simulink model "controller_model_lab_5_R2015"  (R2015a)
settings: Solver=ode5  StartTime=0.0  StopTime=10.0  RelTol=1e-3
values from neighbouring files (symbols this model uses):
  A = [3.98792656502 1 0 0 0 0 -5.81855146071 0 1 0 0 0 ... (36 elements, 6x6)]    [controller_params.mat]    (also in model_params.mat)
  B = [1 0 0 0 0 0]    [controller_params.mat]    (also in model_params.mat)
  C = [-0.000624151634985 0.000754210232314 -7.15793729404e-05 0 0 0]    [controller_params.mat]    (also in model_params.mat)
  D = 0    [controller_params.mat]    (also in model_params.mat)
  DenFilt = [1 -1.6 0.64]    [controller_params.mat]    (also in controller_script.m = poly([alpha alpha]); controller_script_lab_5.m = poly([alpha alpha]))
  kb = compute_strain_constant('plot_collected_data', true, 'plot_selected_data', true)    [compute_constants.m]    (also in compute_strain_constant.m = P(1); controller_params.mat = -7.77292031464; model_params.mat = -7.77292031464)
  Ki_int = -9.9585416323e-05    [controller_params.mat]    (also in controller_script.m = K_int(n_states+1); controller_script_lab_5.m = K_int(n_states+1))
  kp = compute_potentiometer_constant('plot_collected_data', true, 'plot_selected_data', true)    [compute_constants.m]    (also in compute_potentiometer_constant.m = P(1); controller_params.mat = 37.3897251534; model_params.mat = 37.3897251534)
  Kx = [0.00571392119727 -0.0170575156897 0.0161429525348 -0.00224203892548 -0.00421804098625 0.00166256586868]    [controller_params.mat]
  Kx_int = [0.00830854997744 -0.0247918532179 0.023451299358 -0.00325101448541 -0.00612843419234 0.00241434428957]    [controller_params.mat]    (also in controller_script.m = K_int(1:n_states); controller_script_lab_5.m = K_int(1:n_states))
  M = [3543.77501475 3419.31647418 3291.64386704 3161.08265286 3028.02589994 2892.93065581]    [controller_params.mat]
  Nbar = 0.0315325549195    [controller_params.mat]    (also in controller_script.m = Nu + Kx*Nx; controller_script_lab_5.m = Nu + Kx*Nx)
  NumFilt = 0.04    [controller_params.mat]    (also in controller_script.m; controller_script_lab_5.m)
  Ts = 0.001    [controller_params.mat]    (also in controller_script.m; controller_script_lab_5.m)
  x_init = [0 0 0 0 0 0]    [controller_params.mat]    (also in controller_script.m = zeros(n_states, 1); controller_script_lab_5.m = zeros(n_states, 1))
undefined symbols (not defined in the file or in its folder): National_Instruments, PCI
libraries: sldrtlib x3
settings Model: SimulationMode=external  CovHtmlReporting=off  Creator=Alunos  LastModifiedBy=ayesh
settings HardwareCC: ProdBitPerPointer=64  ProdLargestAtomicFloat=Float  ProdIntDivRoundTo=Zero  ProdEndianess=LittleEndian  ProdHWDeviceType=Specified  TargetIntDivRoundTo=Zero  TargetEndianess=LittleEndian  TargetHWDeviceType=Intel->x86/Pentium
settings RTWCC: Description=Simulink Desktop Real-Time  SystemTargetFile=rtwin.tlc  TemplateMakefile=rtwin.tmf  RTWCompilerOptimization=on
settings CodeAppCC: MaxIdLength=95
settings RTWinTargetCC: TargetPreCompLibLocation=C:\Program Files\Polyspace\R2021a\toolbox\sldrt\lib\win64  UseToolchainInfoCompliant=off  ExtModeMexFile=sldrtext

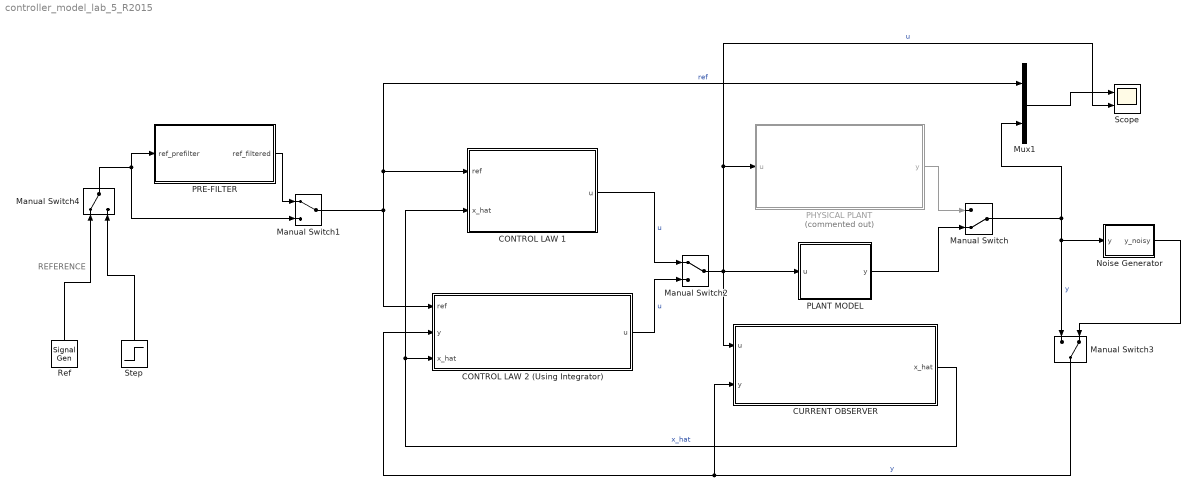
== system controller_model_lab_5_R2015 ==
  note: REFERENCE
  CONTROL LAW 1 : Subsystem
  CONTROL LAW 2 (Using Integrator) : Subsystem
  CURRENT OBSERVER : Subsystem
  Manual Switch : ManualSwitch  CurrentSetting=0
  Manual Switch1 : ManualSwitch
  Manual Switch2 : ManualSwitch
  Manual Switch3 : ManualSwitch  CurrentSetting=0
  Manual Switch4 : ManualSwitch
  Mux1 : Mux  Inputs=2
  Noise Generator : Subsystem
  PHYSICAL PLANT : Subsystem  Commented=on
  PLANT MODEL : Subsystem
  PRE-FILTER : Subsystem
  Ref : SignalGenerator  WaveForm=square  Amplitude=60  Frequency=0.2
  Scope : Scope  NumInputPorts=2
      settings: TimeRange=auto  ShowLegends=on  MaxDataPoints=50000  SaveName=ScopeData  YMin=-75.69471~-4.25511  YMax=75.52983~4.2968  SampleTime=-1
  Step : Step  Time=2  After=30  SampleTime=Ts
  wires:
  Manual Switch2/1 -> Scope/2, PHYSICAL PLANT/1(u), CURRENT OBSERVER/1(u), PLANT MODEL/1(u)  "u"
  Mux1/1 -> Scope/1
  Manual Switch1/1 -> Mux1/1, CONTROL LAW 1/1(ref), CONTROL LAW 2 (Using Integrator)/1(ref)  "ref"
  Manual Switch/1 -> Manual Switch3/1, Noise Generator/1(y), Mux1/2  "y"
  Manual Switch3/1 -> CONTROL LAW 2 (Using Integrator)/2(y), CURRENT OBSERVER/2(y)  "y"
  CURRENT OBSERVER/1(x_hat) -> CONTROL LAW 1/2(x_hat), CONTROL LAW 2 (Using Integrator)/3(x_hat)  "x_hat"
  PLANT MODEL/1(y) -> Manual Switch/2
  PHYSICAL PLANT/1(y) -> Manual Switch/1
  CONTROL LAW 2 (Using Integrator)/1(u) -> Manual Switch2/2  "u"
  CONTROL LAW 1/1(u) -> Manual Switch2/1  "u"
  Noise Generator/1(y_noisy) -> Manual Switch3/2
  Ref/1 -> Manual Switch4/1
  Step/1 -> Manual Switch4/2
  Manual Switch4/1 -> Manual Switch1/2, PRE-FILTER/1(ref_prefilter)
  PRE-FILTER/1(ref_filtered) -> Manual Switch1/1

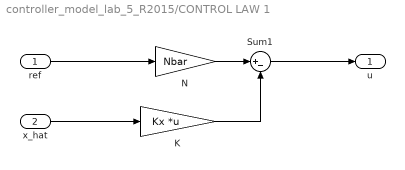
== system controller_model_lab_5_R2015/CONTROL LAW 1 ==
  ref : Inport
  x_hat : Inport  Port=2
  K : Gain  Gain=Kx  Multiplication=Matrix(K*u)
  N : Gain  Gain=Nbar
  Sum1 : Sum  Inputs=|+-
  u : Outport
  wires:
  K/1 -> Sum1/2
  Sum1/1 -> u/1
  N/1 -> Sum1/1
  ref/1 -> N/1
  x_hat/1 -> K/1

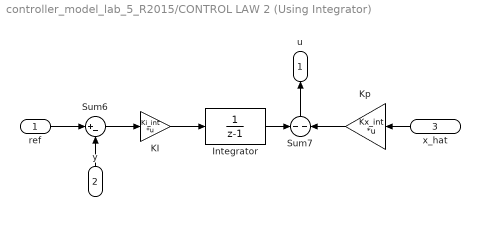
== system controller_model_lab_5_R2015/CONTROL LAW 2 (Using Integrator) ==
  ref : Inport
  y : Inport  Port=2
  x_hat : Inport  Port=3
  Integrator : DiscreteTransferFcn  Denominator=[1 -1]  SampleTime=Ts
  KI : Gain  Gain=Ki_int  Multiplication=Matrix(K*u)
  Kp : Gain  Gain=Kx_int  Multiplication=Matrix(K*u)
  Sum6 : Sum  Inputs=|+-
  Sum7 : Sum  Inputs=--
  u : Outport
  wires:
  y/1 -> Sum6/2
  KI/1 -> Integrator/1
  ref/1 -> Sum6/1
  Sum6/1 -> KI/1
  Integrator/1 -> Sum7/1
  Kp/1 -> Sum7/2
  x_hat/1 -> Kp/1
  Sum7/1 -> u/1

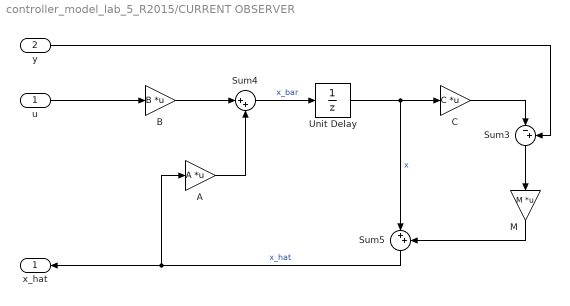
== system controller_model_lab_5_R2015/CURRENT OBSERVER ==
  u : Inport
  y : Inport  Port=2
  A : Gain  Gain=A  Multiplication=Matrix(K*u)
  B : Gain  Gain=B  Multiplication=Matrix(K*u)
  C : Gain  Gain=C  Multiplication=Matrix(K*u)
  M : Gain  Gain=M  Multiplication=Matrix(K*u)
  Sum3 : Sum  Inputs=|-+
  Sum4 : Sum  Inputs=|++
  Sum5 : Sum  Inputs=|++
  Unit Delay : UnitDelay  InitialCondition=x_init  SampleTime=Ts  HasFrameUpgradeWarning=on
  x_hat : Outport
  wires:
  A/1 -> Sum4/2
  Sum4/1 -> Unit Delay/1  "x_bar"
  Unit Delay/1 -> C/1, Sum5/1  "x"
  B/1 -> Sum4/1
  M/1 -> Sum5/2
  C/1 -> Sum3/1
  u/1 -> B/1
  Sum5/1 -> A/1, x_hat/1  "x_hat"
  Sum3/1 -> M/1
  y/1 -> Sum3/2

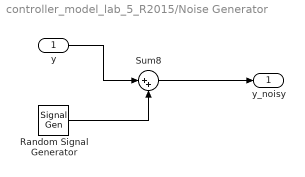
== system controller_model_lab_5_R2015/Noise Generator ==
  y : Inport
  Random Signal Generator : SignalGenerator  WaveForm=random  Amplitude=5  Frequency=0.5
  Sum8 : Sum  Inputs=|++
  y_noisy : Outport
  wires:
  Random Signal Generator/1 -> Sum8/2
  Sum8/1 -> y_noisy/1
  y/1 -> Sum8/1

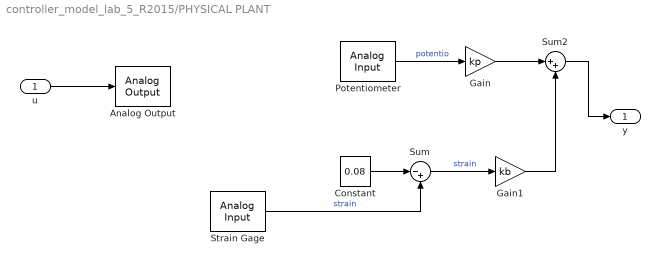
== system controller_model_lab_5_R2015/PHYSICAL PLANT ==
  u : Inport
  Analog Output : sldrtlib/Analog Output  SampleTime=0.001  MaxMissedTicks=10  ShowMissedTicks=off  YieldWhenWaiting=off  DrvName=National_Instruments/PCI-6221  DrvAddress=4294967295  DrvOptions=[0 0 0 0 0]  Channels=1  RangeMode=1  VoltRange=1  InitialValue=0  FinalValue=0
      settings: AttributesFormatString=National Instruments\nPCI-6221 [auto]
  Constant : Constant  Value=0.08
  Gain : Gain  Gain=kp
  Gain1 : Gain  Gain=kb
  Potentiometer : sldrtlib/Analog Input  SampleTime=0.001  MaxMissedTicks=10  ShowMissedTicks=off  YieldWhenWaiting=off  DrvName=National_Instruments/PCI-6221  DrvAddress=4294967295  DrvOptions=[0 0 0 0 0]  Channels=1  RangeMode=1  VoltRange=1  DataType=1
      settings: AttributesFormatString=National Instruments\nPCI-6221 [auto]
  Strain Gage : sldrtlib/Analog Input  SampleTime=0.001  MaxMissedTicks=10  ShowMissedTicks=off  YieldWhenWaiting=off  DrvName=National_Instruments/PCI-6221  DrvAddress=4294967295  DrvOptions=[0 0 0 0 0]  Channels=2  RangeMode=1  VoltRange=1  DataType=1
      settings: AttributesFormatString=National Instruments\nPCI-6221 [auto]
  Sum : Sum  Inputs=|-+
  Sum2 : Sum  Inputs=|++
  y : Outport
  wires:
  Constant/1 -> Sum/1
  Strain Gage/1 -> Sum/2  "strain"
  Potentiometer/1 -> Gain/1  "potentio"
  Gain1/1 -> Sum2/2
  Sum2/1 -> y/1
  Sum/1 -> Gain1/1  "strain"
  Gain/1 -> Sum2/1
  u/1 -> Analog Output/1

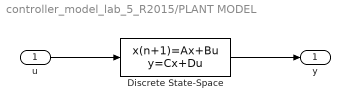
== system controller_model_lab_5_R2015/PLANT MODEL ==
  u : Inport
  Discrete State-Space : DiscreteStateSpace  A=A  B=B  C=C  D=D  X0=x_init  SampleTime=Ts
  y : Outport
  wires:
  u/1 -> Discrete State-Space/1
  Discrete State-Space/1 -> y/1

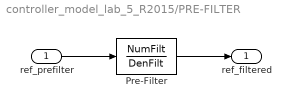
== system controller_model_lab_5_R2015/PRE-FILTER ==
  ref_prefilter : Inport
  Pre-Filter : DiscreteTransferFcn  Numerator=NumFilt  Denominator=DenFilt
  ref_filtered : Outport
  wires:
  ref_prefilter/1 -> Pre-Filter/1
  Pre-Filter/1 -> ref_filtered/1
